simulink model "PN_generator"  (R2020a)
settings: Solver=VariableStepAuto  StartTime=0.0  StopTime=10  RelTol=1e-3
libraries: simulink_extras x1, commutil2 x1, commseqgen3 x1
settings Model: Creator=juanj  LastModifiedBy=juanj

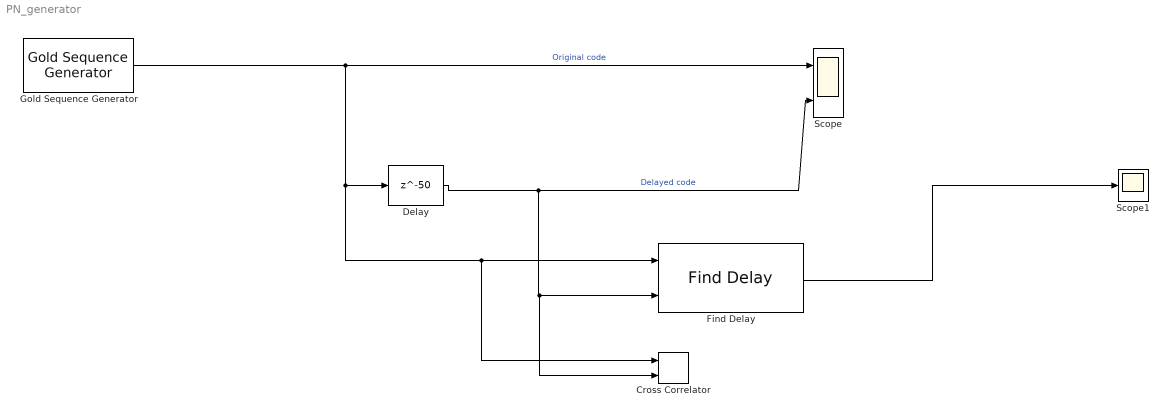
== system PN_generator ==
  Cross Correlator : simulink_extras/Additional Sinks/Cross Correlator  npts=100  HowOften=50  sampleT=1/500
      settings: SourceProductBaseCode=SL
  Delay : Delay  DelayLength=50  InitialCondition=0  UseCircularBuffer=on
  Find Delay : commutil2/Find Delay  corrLength=450  chgSigOP=off  stopUpdate=off  numConstDelay=3
      settings: SourceProductBaseCode=CM
  Gold Sequence Generator : commseqgen3/Gold Sequence Generator  genPoly1='z^6 + z + 1'  iniState1=[0 1 0 1 0 1]  genPoly2='z^6 + z^5 + z^2 + z + 1'  iniState2=[0 0 0 0 0 1]  index=0  shift=0  outVarSiz=off  maxOutSizeMode=Dialog parameter  maxOutSize=[10 1]  Ts=1/500  sampPerFrame=1  reset=off  outDataType=double
      settings: SourceProductBaseCode=CM
  Scope : Scope  NumInputPorts=2
  Scope1 : Scope
  wires:
  Gold Sequence Generator/1 -> Cross Correlator/1, Find Delay/1, Delay/1, Scope/1  "Original code"
  Delay/1 -> Cross Correlator/2, Find Delay/2, Scope/2  "Delayed code"
  Find Delay/1 -> Scope1/1
